simulink model "SecondOrder_nonlinear"  (R2024a)
settings: Solver=VariableStepAuto  StartTime=0.0  StopTime=10  RelTol=1e-3
settings Model: Creator=perruquetti  LastModifiedBy=perruquetti

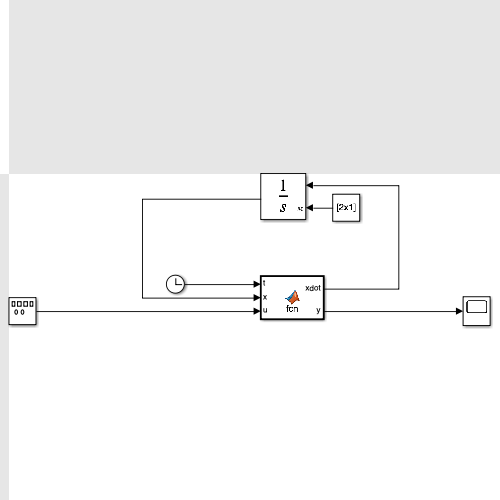
[thumbnail: Simulink's stored preview of the top-level diagram]
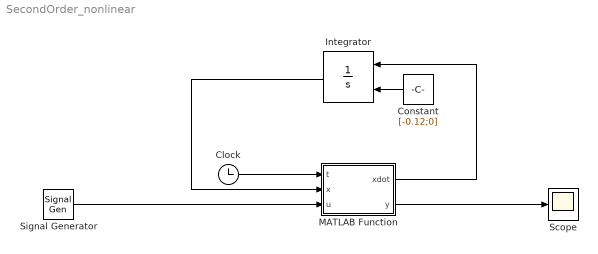
== system SecondOrder_nonlinear ==
  Clock : Clock
  Constant : Constant  Value=[-0.12;0]
  Integrator : Integrator  InitialConditionSource=external  InitialCondition="[-0.12;  0]"
  MATLAB Function : MATLAB Function  TreatAsAtomicUnit=on
  Scope : Scope
  Signal Generator : SignalGenerator  WaveForm=square  Amplitude=0.1  Units=rad/sec
  wires:
  MATLAB Function/1(xdot) -> Integrator/1
  Integrator/1 -> MATLAB Function/2(x)
  MATLAB Function/2(y) -> Scope/1
  Signal Generator/1 -> MATLAB Function/3(u)
  Clock/1 -> MATLAB Function/1(t)
  Constant/1 -> Integrator/2

== matlab function SecondOrder_nonlinear/MATLAB Function ==
  data: t input; x input; xdot output; u input; y output
function [xdot,y] = fcn(t,x,u)
% constants
    a = 2;
%   x1 = -0.12; defined as external IC for the integrator
%   x2 = 0;     
% nonlinear set of equations
    xdot = [x(2)-cos(t)*x(1);
            a*x(1)-x(2)^3+sin(t)*u];
    y = x';
